simulink model "ConventionalVehicleSSC"  (R2026b)
settings: Solver=VariableStepAuto
libraries: fl_lib x1
settings Model: ModifiedByFormat=The MathWorks, Inc.  Creator=The MathWorks, Inc.  LastModifiedBy=The MathWorks, Inc.
settings SimscapeCC: SimscapeUseEnergyAccounting=off

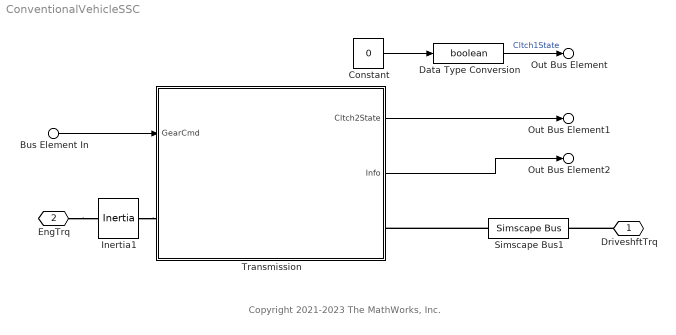
== system ConventionalVehicleSSC ==
  note: Copyright 2021-2023 The MathWorks, Inc.
  Bus Element In : Inport  PortName=Cntrl  Element=Trans.GearCmd
  Constant : Constant  Value=0  SampleTime=Inf
  Data Type Conversion : DataTypeConversion  OutDataTypeStr=boolean  SaturateOnIntegerOverflow=off  RndMeth=Floor
  Inertia1 : fl_lib/Mechanical/Rotational Elements/Inertia  inertia=PlntEngInertia kg*m^2  num_ports=foundation.enum.numPorts2.two  w_specify=off  w_priority=High  w=0 rad/s  w_nominal_specify=off  w_nominal_value=1  w_nominal_unit=rad/s  t_specify=off  t_priority=None  t=0 N*m  t_nominal_specify=off  t_nominal_value=1  t_nominal_unit=N*m
  Simscape Bus1 : SimscapeBus  HierarchyStrings=DriveshftTrq1
  Transmission : Subsystem  Variant=on  VariantControlMode=label  VariantControl=1  LabelModeActiveChoice=Ideal Fixed Gear Transmission
  DriveshftTrq : PMIOPort  Side=Right
  EngTrq : PMIOPort  Port=2  Side=Left
  Out Bus Element : Outport  PortName=TransInfo  Element=Cltch1State
  Out Bus Element1 : Outport  PortName=TransInfo  Element=Cltch2State
  Out Bus Element2 : Outport  PortName=TransInfo  Element=Info
  wires:
  Bus Element In/1 -> Transmission/1(GearCmd)
  Transmission/1(Cltch2State) -> Out Bus Element1/1
  Transmission/2(Info) -> Out Bus Element2/1
  Constant/1 -> Data Type Conversion/1
  Data Type Conversion/1 -> Out Bus Element/1  "Cltch1State"
  connections:
  EngTrq/RConn1 -- Inertia1/RConn1
  Simscape Bus1/LConn1 -- Transmission/RConn1
  Inertia1/LConn1 -- Transmission/LConn1
  DriveshftTrq/RConn1 -- Simscape Bus1/RConn1

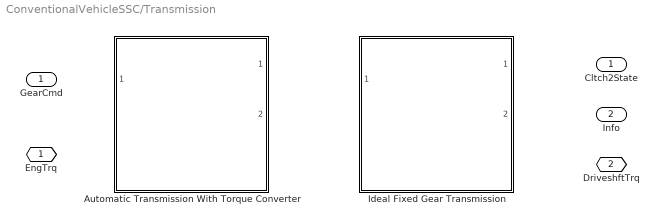
== system ConventionalVehicleSSC/Transmission ==
  GearCmd : Inport
  Automatic Transmission With Torque Converter : Subsystem  VariantControl=Automatic Transmission With Torque Converter  ReferencedSubsystem=AutomaticTransmissionWithTorqueConverterSSC
  Ideal Fixed Gear Transmission : Subsystem  VariantControl=Ideal Fixed Gear Transmission  ReferencedSubsystem=IdealFixedGearTransmissionSSC
  EngTrq : PMIOPort  Side=Left
  DriveshftTrq : PMIOPort  Port=2  Side=Right
  Cltch2State : Outport
  Info : Outport  Port=2
